simulink model "controller"  (Simulink 7.8)
settings: Solver=FixedStepDiscrete  SolverMode=SingleTasking  StartTime=0.0  StopTime=10.0  FixedStep=0.01  RelTol=1e-3
InitFcn:
  | Busses
  | missions
  | common
  | physical_constants
  | l2plus
model workspace: external: MATLAB File (data not in the file)
values from neighbouring files (symbols this model uses):
  InitialPoint = 0    [l2plus.m]
  IPStar = 0    [l2plus.m]
  lla_ltp_gain = [r * (pi / 180 / 1e7); v * cos(ref_lla(1)) * (pi / 180 / 1e7); 1e-6]    [common.m]
  MaxDwnPthStar = 1    [l2plus.m]
  switchDistance = 4    [l2plus.m]
  T_step = 0.01    [common.m]
  tanIntercept = tan( 45*pi/180 )    [l2plus.m]
  TStar = single(2)    [l2plus.m]
  Turn2Track = 0    [l2plus.m]
  wheelbase = 3.27    [physical_constants.m]
undefined symbols (not defined in the file or in its folder): DiscIntNeverNeededParam, gps_offset, GpsOffsetCorrectionEnable, gpsOrigin, KPsiDot, test_waypoints
libraries: uSimLib x16, aerolibutil x2, aerolibtransform2 x1
settings Model: Creator=bwmairs  LastModifiedBy=Bryant
settings DataIOCC: SignalLogging=off  DSMLogging=off
settings OptimizationCC: BlockReduction=off  InlineParams=on  InlineInvariantSignals=on  PassReuseOutputArgsAs=Individual arguments  ZeroExternalMemoryAtStartup=off  ZeroInternalMemoryAtStartup=off  InitFltsAndDblsToZero=on  NoFixptDivByZeroProtection=on  EfficientFloat2IntCast=on  OptimizeModelRefInitCode=on  LifeSpan=30
settings DebuggingCC: ReadBeforeWriteMsg=DisableAll  WriteAfterWriteMsg=DisableAll  WriteAfterReadMsg=DisableAll  UnderspecifiedInitializationDetection=Simplified  ParameterOverflowMsg=warning  FcnCallInpInsideContextMsg=Use local settings  UniqueDataStoreMsg=error
settings HardwareCC: ProdHWDeviceType=Generic->Unspecified (assume 32-bit Generic)  TargetBitPerInt=16  TargetBitPerPointer=16  TargetIntDivRoundTo=Zero  TargetEndianess=LittleEndian  TargetWordSize=16  TargetHWDeviceType=Microchip->dsPIC  ProdEqTarget=off
settings ModelReferenceCC: ModelReferenceNumInstancesAllowed=Single
settings SFSimCC: SimCustomHeaderCode="#include \"Missions.h\""  SimUserIncludeDirs=../Libs/C  SimParseCustomCode=off
settings RTWCC: SystemTargetFile=ert.tlc  GenCodeOnly=on  GenerateMakefile=off  TemplateMakefile=ert_default_tmf  Description=Embedded Coder  ProcessScript=ert_make_rtw_hook  RTWCompilerOptimization=On
settings CodeAppCC: IgnoreCustomStorageClasses=off  IgnoreTestpoints=on
settings ERTTargetCC: MultiwordLength=2048  IncludeMdlTerminateFcn=off  SupportComplex=off  InlinedParameterPlacement=NonHierarchical  ERTCustomFileTemplate=example_file_process.tlc  ConvertIfToSwitch=off  SuppressUnreachableDefaultCases=off

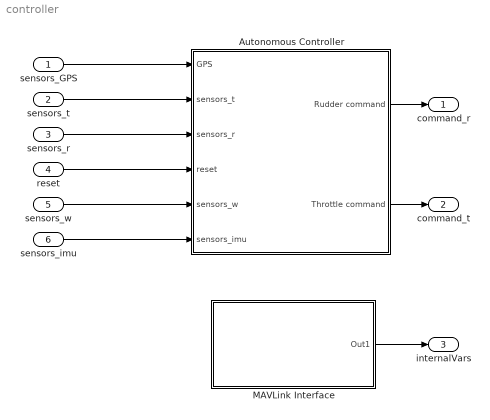
== system controller ==
  sensors_GPS : Inport  OutDataTypeStr=Bus: GpsData  PortDimensions=1
  sensors_t : Inport  Port=2  OutDataTypeStr=int16  PortDimensions=1
  sensors_r : Inport  Port=3  OutDataTypeStr=single  PortDimensions=1
  reset : Inport  Port=4  OutDataTypeStr=boolean  PortDimensions=1
  sensors_w : Inport  Port=5  OutDataTypeStr=single  PortDimensions=1
  sensors_imu : Inport  Port=6  OutDataTypeStr=Bus: ImuData  PortDimensions=1
  Autonomous Controller : Subsystem  Priority=1
  MAVLink Interface : Subsystem
  command_r : Outport  OutDataTypeStr=single  PortDimensions=1
  command_t : Outport  Port=2  OutDataTypeStr=int16  PortDimensions=1
  internalVars : Outport  Port=3  OutDataTypeStr=Bus: InternalVariables  PortDimensions=1
  wires:
  sensors_t/1 -> Autonomous Controller/2(sensors_t)
  sensors_GPS/1 -> Autonomous Controller/1(GPS)
  reset/1 -> Autonomous Controller/4(reset)
  sensors_r/1 -> Autonomous Controller/3(sensors_r)
  Autonomous Controller/2(Throttle command) -> command_t/1
  Autonomous Controller/1(Rudder command) -> command_r/1
  sensors_w/1 -> Autonomous Controller/5(sensors_w)
  MAVLink Interface/1(Out1) -> internalVars/1
  sensors_imu/1 -> Autonomous Controller/6(sensors_imu)

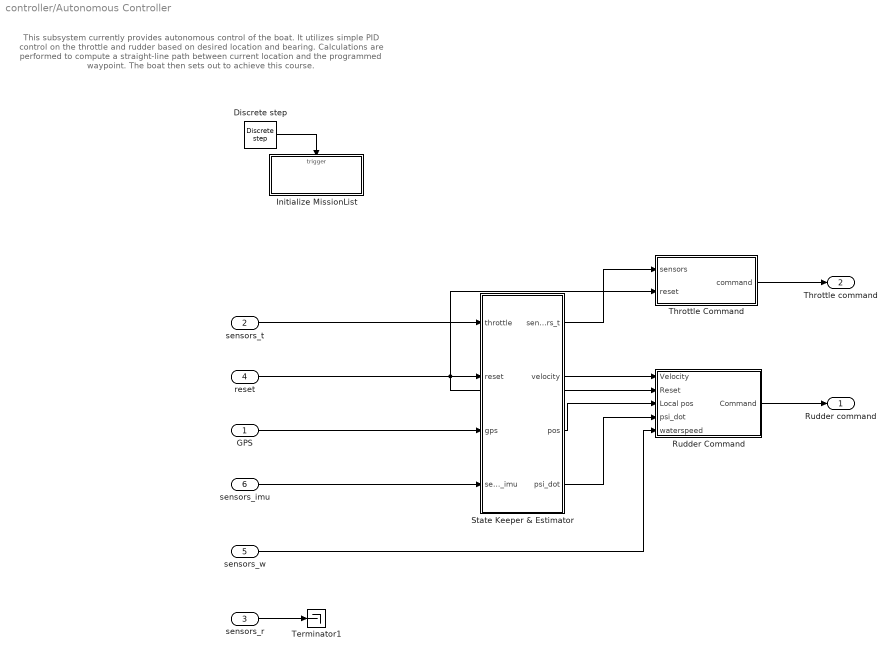
== system controller/Autonomous Controller ==
  note: This subsystem currently provides autonomous control of the boat. It utilizes simple PID control
      | on the throttle and rudder based on desired location and bearing. Calculations are performed
      | to compute a straight-line path between current location and the programmed waypoint. The
      | boat then sets out to achieve this course.
  GPS : Inport
  sensors_t : Inport  Port=2
  sensors_r : Inport  Port=3
  reset : Inport  Port=4
  sensors_w : Inport  Port=5
  sensors_imu : Inport  Port=6
  Discrete step : uSimLib/Sources/Discrete step  start_value=1  end_value=0  transition_time=1
  Initialize MissionList : Subsystem  TreatAsAtomicUnit=on
  Rudder Command : Subsystem
  State Keeper & Estimator : Subsystem
  Terminator1 : Terminator
  Throttle Command : Subsystem
  Rudder command : Outport
  Throttle command : Outport  Port=2
  wires:
  Discrete step/1 -> Initialize MissionList/Trigger
  reset/1 -> Rudder Command/2(Reset), Throttle Command/2(reset), State Keeper & Estimator/2(reset)
  State Keeper & Estimator/3(pos) -> Rudder Command/3(Local pos)
  State Keeper & Estimator/1(sensors_t) -> Throttle Command/1(sensors)
  State Keeper & Estimator/2(velocity) -> Rudder Command/1(Velocity)
  GPS/1 -> State Keeper & Estimator/3(gps)
  Throttle Command/1(command) -> Throttle command/1
  Rudder Command/1(Command) -> Rudder command/1
  sensors_r/1 -> Terminator1/1
  sensors_t/1 -> State Keeper & Estimator/1(throttle)
  State Keeper & Estimator/4(psi_dot) -> Rudder Command/4(psi_dot)
  sensors_w/1 -> Rudder Command/5(waterspeed)
  sensors_imu/1 -> State Keeper & Estimator/4(sensors_imu)

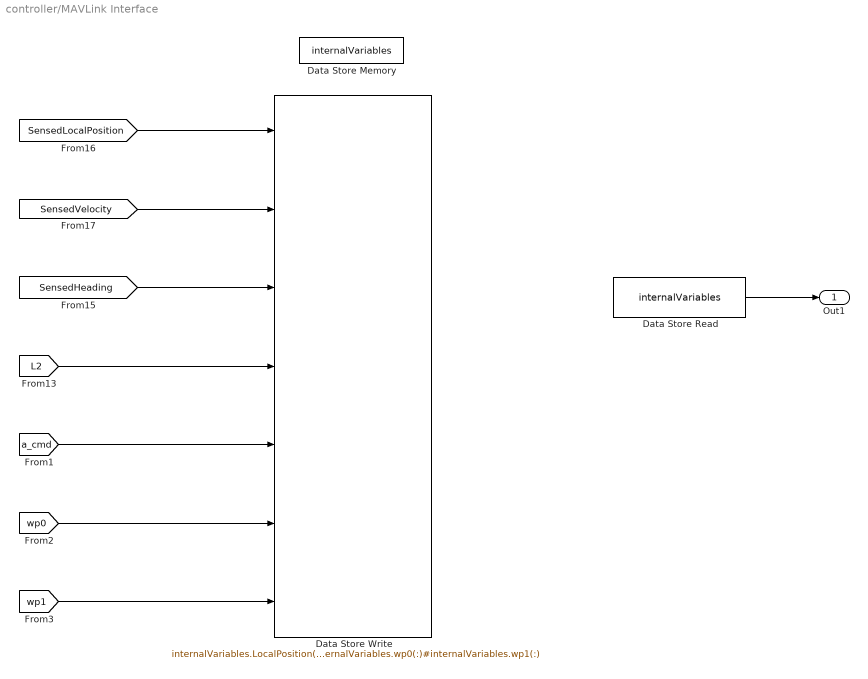
== system controller/MAVLink Interface ==
  Data Store Memory : DataStoreMemory  DataStoreName=internalVariables  OutDataTypeStr=Bus: InternalVariables
  Data Store Read : DataStoreRead  DataStoreName=internalVariables  SampleTime=T_step  DataStoreElements=internalVariables
  Data Store Write : DataStoreWrite  DataStoreName=internalVariables  DataStoreElements=internalVariables.LocalPosition(:)#internalVariables.Velocity(:)#internalVariables.Heading#internalVariables.L2Vector(:)#internalVariables.Acmd#internalVariables.wp0(:)#internalVariables.wp1(:)
  Out1 : Outport  OutDataTypeStr=Bus: InternalVariables
  wires:
  [SensedLocalPosition] -> Data Store Write/1
  [SensedVelocity] -> Data Store Write/2
  [SensedHeading] -> Data Store Write/3
  [L2] -> Data Store Write/4
  [a_cmd] -> Data Store Write/5
  [wp0] -> Data Store Write/6
  [wp1] -> Data Store Write/7
  Data Store Read/1 -> Out1/1

== system controller/Autonomous Controller/Initialize MissionList ==
  Trigger : TriggerPort  TriggerType=falling  PortDimensions=1
  AppendMission : uSimLib/Mission Manager/AppendMission  Priority=-2  sampleTime=-1
  ClearMissionList : uSimLib/Mission Manager/ClearMissionList  Priority=-1  sampleTime=-1
  Constant : Constant  Value=test_waypoints(1)  OutDataTypeStr=Bus: Mission
  Data Type Conversion : DataTypeConversion  OutDataTypeStr=uint8  RndMeth=Simplest
  Mission Init : uSimLib/Mission Manager/Mission Init  Priority=-3  maxMissions=16  sampleTime=-1
  Mission InitAll : uSimLib/Mission Manager/Mission InitAll  Priority=0  maxMissions=16  sampleTime=-1  missionsVar=test_waypoints
  SetCurrentMission : uSimLib/Mission Manager/SetCurrentMission  sampleTime=-1
  wires:
  AppendMission/1 -> Data Type Conversion/1
  Constant/1 -> AppendMission/1
  Data Type Conversion/1 -> SetCurrentMission/1

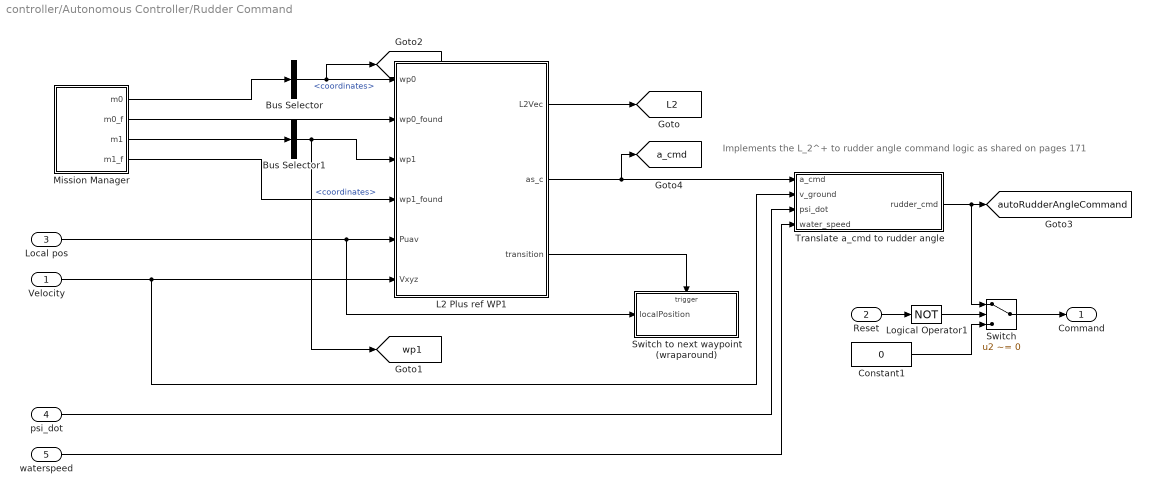
== system controller/Autonomous Controller/Rudder Command ==
  note: Implements the L_2^+ to rudder angle command logic as shared on pages 171
  Velocity : Inport
  Reset : Inport  Port=2
  Local pos : Inport  Port=3
  psi_dot : Inport  Port=4
  waterspeed : Inport  Port=5
  Bus Selector : BusSelector  OutputSignals=coordinates
  Bus Selector1 : BusSelector  OutputSignals=coordinates
  Constant1 : Constant  Value=0  OutDataTypeStr=single
  L2 Plus ref WP1 : MATLAB Function  TreatAsAtomicUnit=on
  Logical Operator1 : Logic  Operator=NOT  Inputs=1  AllPortsSameDT=off  OutDataTypeStr=boolean
  Mission Manager : Subsystem
  Switch : Switch  Criteria=u2 ~= 0
  Switch to next waypoint (wraparound) : Subsystem  TreatAsAtomicUnit=on
  Translate a_cmd to rudder angle : Subsystem
  Command : Outport
  tag scope: L2=global, a_cmd=global, autoRudderAngleCommand=global, wp0=global, wp1=global
  wires:
  Bus Selector1/1 -> L2 Plus ref WP1/3(wp1), [wp1]  "<coordinates>"
  Bus Selector/1 -> [wp0], L2 Plus ref WP1/1(wp0)  "<coordinates>"
  Mission Manager/1(m0) -> Bus Selector/1
  Mission Manager/2(m0_f) -> L2 Plus ref WP1/2(wp0_found)
  L2 Plus ref WP1/3(transition) -> Switch to next waypoint (wraparound)/Trigger
  Mission Manager/4(m1_f) -> L2 Plus ref WP1/4(wp1_found)
  Mission Manager/3(m1) -> Bus Selector1/1
  Local pos/1 -> Switch to next waypoint (wraparound)/1(localPosition), L2 Plus ref WP1/5(Puav)
  Velocity/1 -> L2 Plus ref WP1/6(Vxyz), Translate a_cmd to rudder angle/2(v_ground)
  L2 Plus ref WP1/1(L2Vec) -> [L2]
  Translate a_cmd to rudder angle/1(rudder_cmd) -> [autoRudderAngleCommand], Switch/1
  Reset/1 -> Logical Operator1/1
  Logical Operator1/1 -> Switch/2
  L2 Plus ref WP1/2(as_c) -> [a_cmd], Translate a_cmd to rudder angle/1(a_cmd)
  psi_dot/1 -> Translate a_cmd to rudder angle/3(psi_dot)
  waterspeed/1 -> Translate a_cmd to rudder angle/4(water_speed)
  Constant1/1 -> Switch/3
  Switch/1 -> Command/1

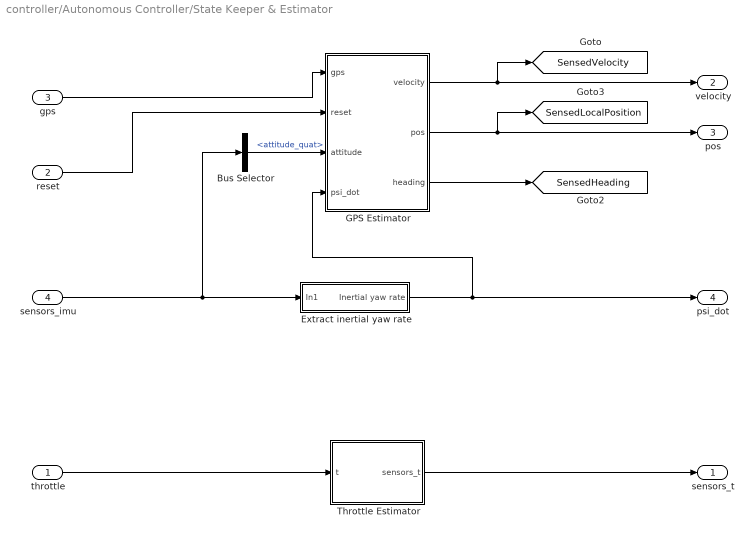
== system controller/Autonomous Controller/State Keeper & Estimator ==
  throttle : Inport
  reset : Inport  Port=2
  gps : Inport  Port=3
  sensors_imu : Inport  Port=4
  Bus Selector : BusSelector  OutputSignals=attitude_quat
  Extract inertial yaw rate : Subsystem
  GPS Estimator : Subsystem
  Throttle Estimator : Subsystem
  sensors_t : Outport
  velocity : Outport  Port=2
  pos : Outport  Port=3
  psi_dot : Outport  Port=4
  tag scope: SensedHeading=global, SensedLocalPosition=global, SensedVelocity=global
  wires:
  Throttle Estimator/1(sensors_t) -> sensors_t/1
  GPS Estimator/3(heading) -> [SensedHeading]
  GPS Estimator/2(pos) -> [SensedLocalPosition], pos/1
  gps/1 -> GPS Estimator/1(gps)
  GPS Estimator/1(velocity) -> [SensedVelocity], velocity/1
  reset/1 -> GPS Estimator/2(reset)
  throttle/1 -> Throttle Estimator/1(t)
  sensors_imu/1 -> Extract inertial yaw rate/1(In1), Bus Selector/1
  Extract inertial yaw rate/1(Inertial yaw rate) -> psi_dot/1, GPS Estimator/4(psi_dot)
  Bus Selector/1 -> GPS Estimator/3(attitude)  "<attitude_quat>"

== system controller/Autonomous Controller/Throttle Command ==
  sensors : Inport
  reset : Inport  Port=2
  Constant1 : Constant  Value=0  OutDataTypeStr=int16
  Constant5 : Constant  Value=1000  OutDataTypeStr=int16
  Switch : Switch  Criteria=u2 > Threshold
  Terminator : Terminator
  command : Outport
  tag scope: autoThrottleCommand=global
  wires:
  Constant5/1 -> Switch/3
  Constant1/1 -> Switch/1
  reset/1 -> Switch/2
  sensors/1 -> Terminator/1
  Switch/1 -> [autoThrottleCommand], command/1

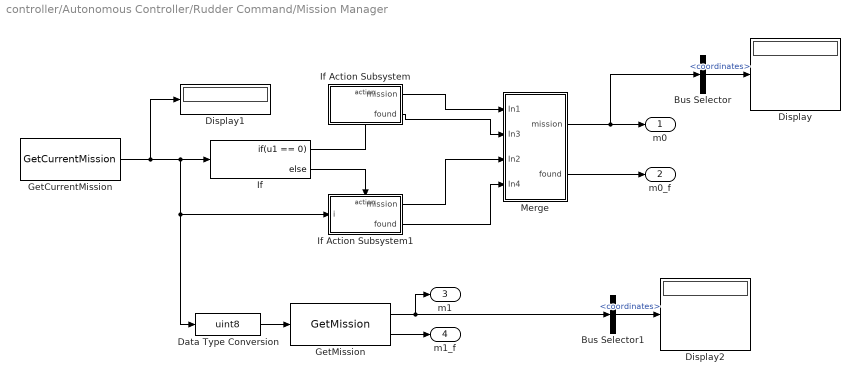
== system controller/Autonomous Controller/Rudder Command/Mission Manager ==
  Bus Selector : BusSelector  OutputSignals=coordinates
  Bus Selector1 : BusSelector  OutputSignals=coordinates
  Data Type Conversion : DataTypeConversion  OutDataTypeStr=uint8
  Display : Display
  Display1 : Display
  Display2 : Display
  GetCurrentMission : uSimLib/Mission Manager/GetCurrentMission  sampleTime=T_step
  GetMission : uSimLib/Mission Manager/GetMission  sampleTime=T_step
  If : If  IfExpression=u1 == 0
  If Action Subsystem : Subsystem  TreatAsAtomicUnit=on
  If Action Subsystem1 : Subsystem  TreatAsAtomicUnit=on
  Merge : Subsystem
  m0 : Outport
  m0_f : Outport  Port=2
  m1 : Outport  Port=3
  m1_f : Outport  Port=4
  wires:
  Data Type Conversion/1 -> GetMission/1
  Merge/2(found) -> m0_f/1
  Merge/1(mission) -> m0/1, Bus Selector/1
  If Action Subsystem1/2(found) -> Merge/4(In4)
  If Action Subsystem/2(found) -> Merge/2(In3)
  If Action Subsystem1/1(mission) -> Merge/3(In2)
  If Action Subsystem/1(mission) -> Merge/1(In1)
  If/2 -> If Action Subsystem1/Action
  If/1 -> If Action Subsystem/Action
  GetMission/2 -> m1_f/1
  GetMission/1 -> m1/1, Bus Selector1/1
  GetCurrentMission/1 -> If/1, Data Type Conversion/1, If Action Subsystem1/1(i), Display1/1
  Bus Selector/1 -> Display/1  "<coordinates>"
  Bus Selector1/1 -> Display2/1  "<coordinates>"

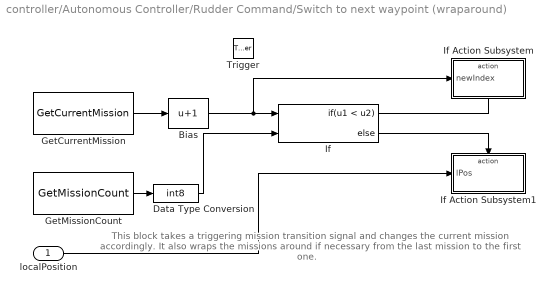
== system controller/Autonomous Controller/Rudder Command/Switch to next waypoint (wraparound) ==
  note: This block takes a triggering mission transition signal
      | and changes the current mission accordingly. It also
      | wraps the missions around if necessary from the last
      | mission to the first one.
  localPosition : Inport
  Trigger : TriggerPort
  Bias : Bias  Bias=1
  Data Type Conversion : DataTypeConversion  OutDataTypeStr=int8
  GetCurrentMission : uSimLib/Mission Manager/GetCurrentMission  sampleTime=-1
  GetMissionCount : uSimLib/Mission Manager/GetMissionCount  sampleTime=-1
  If : If  NumInputs=2  IfExpression=u1 < u2
  If Action Subsystem : Subsystem  TreatAsAtomicUnit=on
  If Action Subsystem1 : Subsystem  TreatAsAtomicUnit=on
  wires:
  Data Type Conversion/1 -> If/2
  If/2 -> If Action Subsystem1/Action
  If/1 -> If Action Subsystem/Action
  Bias/1 -> If/1, If Action Subsystem/1(newIndex)
  GetMissionCount/1 -> Data Type Conversion/1
  GetCurrentMission/1 -> Bias/1
  localPosition/1 -> If Action Subsystem1/1(lPos)

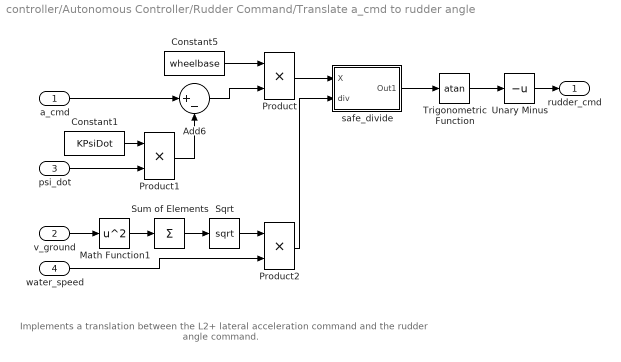
== system controller/Autonomous Controller/Rudder Command/Translate a_cmd to rudder angle ==
  note: Implements a translation between the L2+ lateral acceleration command
      | and the rudder angle command.
  a_cmd : Inport
  v_ground : Inport  Port=2
  psi_dot : Inport  Port=3
  water_speed : Inport  Port=4
  Add6 : Sum  Inputs=|+-
  Constant1 : Constant  Value=KPsiDot
  Constant5 : Constant  Value=wheelbase
  Math Function1 : Math  Operator=square  SaturateOnIntegerOverflow=on
  Product : Product  Inputs=**  RndMeth=Zero
  Product1 : Product  Inputs=**  RndMeth=Zero
  Product2 : Product  Inputs=**  RndMeth=Zero
  Sqrt : Sqrt  SaturateOnIntegerOverflow=on
  Sum of Elements : Sum  Inputs=+
  Trigonometric Function : Trigonometry  Operator=atan
  Unary Minus : UnaryMinus
  safe_divide : Subsystem  TreatAsAtomicUnit=on
      settings: RTWFcnNameOpts=Use subsystem name  RTWFileNameOpts=Use function name
  rudder_cmd : Outport
  wires:
  Constant5/1 -> Product/1
  Product/1 -> safe_divide/1(X)
  Trigonometric Function/1 -> Unary Minus/1
  Math Function1/1 -> Sum of Elements/1
  Sum of Elements/1 -> Sqrt/1
  safe_divide/1(Out1) -> Trigonometric Function/1
  Add6/1 -> Product/2
  v_ground/1 -> Math Function1/1
  Unary Minus/1 -> rudder_cmd/1
  a_cmd/1 -> Add6/1
  psi_dot/1 -> Product1/2
  Constant1/1 -> Product1/1
  Sqrt/1 -> Product2/1
  Product2/1 -> safe_divide/2(div)
  water_speed/1 -> Product2/2
  Product1/1 -> Add6/2

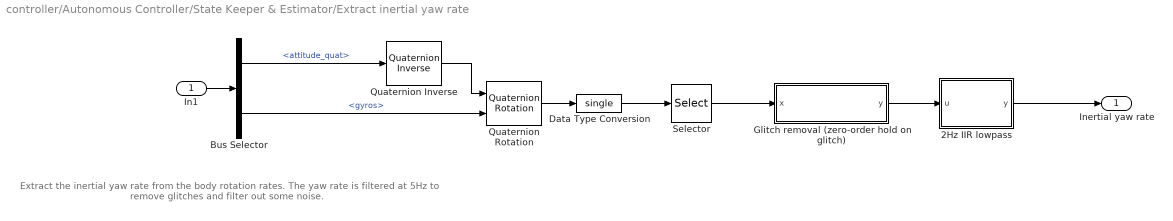
== system controller/Autonomous Controller/State Keeper & Estimator/Extract inertial yaw rate ==
  note: Extract the inertial yaw rate from the body rotation rates.
      | The yaw rate is filtered at 5Hz to remove glitches and filter out some noise.
  In1 : Inport
  2Hz IIR lowpass : MATLAB Function  TreatAsAtomicUnit=on
  Bus Selector : BusSelector  OutputSignals=attitude_quat,gyros
  Data Type Conversion : DataTypeConversion  OutDataTypeStr=single
  Glitch removal (zero-order hold on glitch) : MATLAB Function  TreatAsAtomicUnit=on
  Quaternion Inverse : aerolibutil/Quaternion Inverse
  Quaternion Rotation : aerolibutil/Quaternion Rotation
  Selector : Selector  InputPortWidth=3  IndexOptions=Index vector (dialog)  Indices=[3]  OutputSizes=1
  Inertial yaw rate : Outport
  wires:
  In1/1 -> Bus Selector/1
  Quaternion Inverse/1 -> Quaternion Rotation/1
  Quaternion Rotation/1 -> Data Type Conversion/1
  Data Type Conversion/1 -> Selector/1
  Selector/1 -> Glitch removal (zero-order hold on glitch)/1(x)
  Glitch removal (zero-order hold on glitch)/1(y) -> 2Hz IIR lowpass/1(u)
  Bus Selector/2 -> Quaternion Rotation/2  "<gyros>"
  2Hz IIR lowpass/1(y) -> Inertial yaw rate/1
  Bus Selector/1 -> Quaternion Inverse/1  "<attitude_quat>"

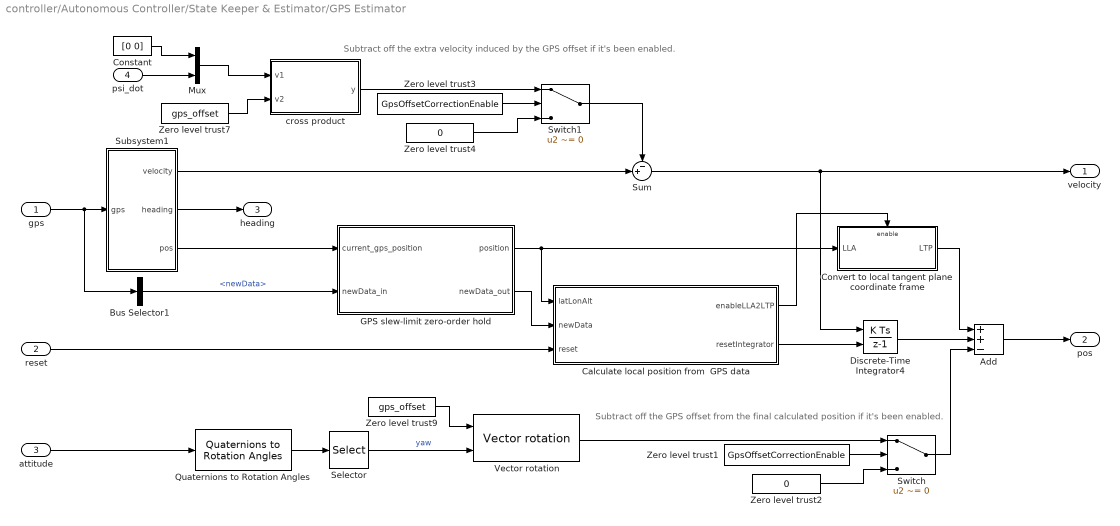
== system controller/Autonomous Controller/State Keeper & Estimator/GPS Estimator ==
  note: Subtract off the GPS offset from the final calculated position if it's
      | been enabled.
  note: Subtract off the extra velocity induced by the GPS offset
      | if it's been enabled.
  gps : Inport
  reset : Inport  Port=2
  attitude : Inport  Port=3
  psi_dot : Inport  Port=4  OutDataTypeStr=single
  Add : Sum  Inputs=++-
  Bus Selector1 : BusSelector  OutputSignals=newData
  Calculate local position from  GPS data : MATLAB Function  TreatAsAtomicUnit=on
  Constant : Constant  Value=[0 0]  OutDataTypeStr=single
  Convert to local tangent plane coordinate frame : Subsystem  TreatAsAtomicUnit=on  RTWFcnName=lla2ltp
      settings: RTWFcnNameOpts=User specified
  Discrete-Time Integrator4 : DiscreteIntegrator  ExternalReset=level  SampleTime=-1  ICPrevOutput=DiscIntNeverNeededParam  ICPrevScaledInput=DiscIntNeverNeededParam
  GPS slew-limit zero-order hold : MATLAB Function  TreatAsAtomicUnit=on
  Mux : Mux  Inputs=2
  Quaternions to Rotation Angles : aerolibtransform2/Quaternions to Rotation Angles  rotationOrder=ZYX
  Selector : Selector  InputPortWidth=3  IndexOptions=Index vector (dialog)  Indices=[1]  OutputSizes=1
  Subsystem1 : Subsystem
  Sum : Sum  Inputs=-+|
  Switch : Switch  Criteria=u2 ~= 0  OutDataTypeStr=Inherit: Inherit via back propagation  RndMeth=Simplest
  Switch1 : Switch  Criteria=u2 ~= 0  OutDataTypeStr=Inherit: Inherit via back propagation  RndMeth=Simplest
  Vector rotation : uSimLib/Math/Vector rotation
  Zero level trust1 : Constant  Value=GpsOffsetCorrectionEnable  OutDataTypeStr=boolean
  Zero level trust2 : Constant  Value=0  OutDataTypeStr=single
  Zero level trust3 : Constant  Value=GpsOffsetCorrectionEnable  OutDataTypeStr=boolean
  Zero level trust4 : Constant  Value=0  OutDataTypeStr=single
  Zero level trust7 : Constant  Value=gps_offset  OutDataTypeStr=single
  Zero level trust9 : Constant  Value=gps_offset  OutDataTypeStr=single
  cross product : MATLAB Function  TreatAsAtomicUnit=on
  velocity : Outport
  pos : Outport  Port=2
  heading : Outport  Port=3
  wires:
  Calculate local position from  GPS data/2(resetIntegrator) -> Discrete-Time Integrator4/2
  Add/1 -> pos/1
  Discrete-Time Integrator4/1 -> Add/2
  Subsystem1/3(pos) -> GPS slew-limit zero-order hold/1(current_gps_position)
  gps/1 -> Bus Selector1/1, Subsystem1/1(gps)
  Subsystem1/2(heading) -> heading/1
  reset/1 -> Calculate local position from  GPS data/3(reset)
  Convert to local tangent plane coordinate frame/1(LTP) -> Add/1
  Calculate local position from  GPS data/1(enableLLA2LTP) -> Convert to local tangent plane coordinate frame/Enable
  GPS slew-limit zero-order hold/1(position) -> Calculate local position from  GPS data/1(latLonAlt), Convert to local tangent plane coordinate frame/1(LLA)
  GPS slew-limit zero-order hold/2(newData_out) -> Calculate local position from  GPS data/2(newData)
  Bus Selector1/1 -> GPS slew-limit zero-order hold/2(newData_in)  "<newData>"
  attitude/1 -> Quaternions to Rotation Angles/1
  Quaternions to Rotation Angles/1 -> Selector/1
  Constant/1 -> Mux/1
  psi_dot/1 -> Mux/2
  Zero level trust7/1 -> cross product/2(v2)
  Mux/1 -> cross product/1(v1)
  Subsystem1/1(velocity) -> Sum/2
  Sum/1 -> Discrete-Time Integrator4/1, velocity/1
  Selector/1 -> Vector rotation/2  "yaw"
  Zero level trust9/1 -> Vector rotation/1
  cross product/1(y) -> Switch1/1
  Switch/1 -> Add/3
  Zero level trust1/1 -> Switch/2
  Vector rotation/1 -> Switch/1
  Zero level trust2/1 -> Switch/3
  Zero level trust3/1 -> Switch1/2
  Zero level trust4/1 -> Switch1/3
  Switch1/1 -> Sum/1

== system controller/Autonomous Controller/State Keeper & Estimator/Throttle Estimator ==
  t : Inport
  sensors_t : Outport
  wires:
  t/1 -> sensors_t/1

== system controller/Autonomous Controller/Rudder Command/Mission Manager/If Action Subsystem ==
  Action Port : ActionPort  ActionType=then
  Constant : Constant  Value=true  OutDataTypeStr=boolean
  GetStartingPoint : uSimLib/Mission Manager/GetStartingPoint  sampleTime=-1
  mission : Outport
  found : Outport  Port=2
  wires:
  Constant/1 -> found/1
  GetStartingPoint/1 -> mission/1

== system controller/Autonomous Controller/Rudder Command/Mission Manager/If Action Subsystem1 ==
  i : Inport
  Action Port : ActionPort  ActionType=else
  Bias : Bias  Bias=-1
  Data Type Conversion : DataTypeConversion  OutDataTypeStr=uint8
  GetMission : uSimLib/Mission Manager/GetMission  sampleTime=-1
  mission : Outport
  found : Outport  Port=2
  wires:
  Data Type Conversion/1 -> GetMission/1
  Bias/1 -> Data Type Conversion/1
  GetMission/2 -> found/1
  i/1 -> Bias/1
  GetMission/1 -> mission/1

== system controller/Autonomous Controller/Rudder Command/Mission Manager/Merge ==
  In1 : Inport
  In3 : Inport  Port=2
  In2 : Inport  Port=3
  In4 : Inport  Port=4
  Merge : Merge
  Merge1 : Merge
  mission : Outport
  found : Outport  Port=2
  wires:
  In4/1 -> Merge1/2
  Merge1/1 -> found/1
  In3/1 -> Merge1/1
  In2/1 -> Merge/2
  Merge/1 -> mission/1
  In1/1 -> Merge/1

== system controller/Autonomous Controller/Rudder Command/Switch to next waypoint (wraparound)/If Action Subsystem ==
  newIndex : Inport
  Action Port : ActionPort  ActionType=then
  Data Type Conversion : DataTypeConversion  OutDataTypeStr=uint8
  SetCurrentMission : uSimLib/Mission Manager/SetCurrentMission  sampleTime=-1
  wires:
  Data Type Conversion/1 -> SetCurrentMission/1
  newIndex/1 -> Data Type Conversion/1

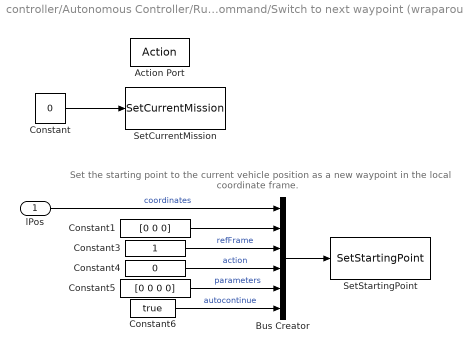
== system controller/Autonomous Controller/Rudder Command/Switch to next waypoint (wraparound)/If Action Subsystem1 ==
  note: Set the starting point to the current vehicle position as a new waypoint in the local coordinate frame.
  lPos : Inport
  Action Port : ActionPort  ActionType=else
  Bus Creator : BusCreator  Inputs=6  OutDataTypeStr=Bus: Mission  NonVirtualBus=on
  Constant : Constant  Value=0  OutDataTypeStr=uint8
  Constant1 : Constant  Value=[0 0 0]  OutDataTypeStr=single
  Constant3 : Constant  OutDataTypeStr=uint8
  Constant4 : Constant  Value=0  OutDataTypeStr=uint8
  Constant5 : Constant  Value=[0 0 0 0]  OutDataTypeStr=single
  Constant6 : Constant  Value=true  OutDataTypeStr=boolean
  SetCurrentMission : uSimLib/Mission Manager/SetCurrentMission  sampleTime=-1
  SetStartingPoint : uSimLib/Mission Manager/SetStartingPoint  sampleTime=-1
  wires:
  Constant/1 -> SetCurrentMission/1
  Constant6/1 -> Bus Creator/6  "autocontinue"
  Constant5/1 -> Bus Creator/5  "parameters"
  Constant4/1 -> Bus Creator/4  "action"
  Constant3/1 -> Bus Creator/3  "refFrame"
  lPos/1 -> Bus Creator/1  "coordinates"
  Bus Creator/1 -> SetStartingPoint/1
  Constant1/1 -> Bus Creator/2

== system controller/Autonomous Controller/Rudder Command/Translate a_cmd to rudder angle/safe_divide ==
  X : Inport
  div : Inport  Port=2
  Constant1 : Constant  Value=0  OutDataTypeStr=Inherit: Inherit via back propagation
  Product : Product  Inputs=*/  RndMeth=Zero
  Switch : Switch  Criteria=u2 ~= 0
  Out1 : Outport
  wires:
  X/1 -> Product/1
  div/1 -> Product/2, Switch/2
  Product/1 -> Switch/1
  Constant1/1 -> Switch/3
  Switch/1 -> Out1/1

== system controller/Autonomous Controller/State Keeper & Estimator/GPS Estimator/Convert to local tangent plane coordinate frame ==
  LLA : Inport
  Enable : EnablePort
  LLA2LTP : Subsystem  TreatAsAtomicUnit=on  RTWFcnName=lla2ltp
      settings: RTWFcnNameOpts=User specified
  LTP : Outport  OutDataTypeStr=single  InitialOutput=[0, 0, 0]
  wires:
  LLA/1 -> LLA2LTP/1(LLA)
  LLA2LTP/1(LTP) -> LTP/1

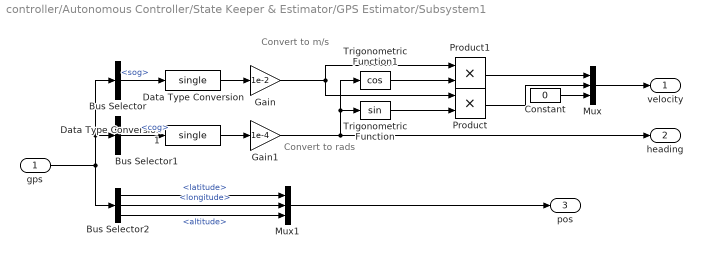
== system controller/Autonomous Controller/State Keeper & Estimator/GPS Estimator/Subsystem1 ==
  note: Convert to m/s
  note: Convert to rads
  gps : Inport
  Bus Selector : BusSelector  OutputSignals=sog
  Bus Selector1 : BusSelector  OutputSignals=cog
  Bus Selector2 : BusSelector  OutputSignals=latitude,longitude,altitude
  Constant : Constant  Value=0  OutDataTypeStr=single
  Data Type Conversion : DataTypeConversion  OutDataTypeStr=single  RndMeth=Simplest
  Data Type Conversion1 : DataTypeConversion  OutDataTypeStr=single  RndMeth=Simplest
  Gain : Gain  Gain=1e-2
  Gain1 : Gain  Gain=1e-4
  Mux : Mux  Inputs=3
  Mux1 : Mux  Inputs=3
  Product : Product  OutDataTypeStr=single  RndMeth=Zero
  Product1 : Product  OutDataTypeStr=single  RndMeth=Zero
  Trigonometric Function : Trigonometry
  Trigonometric Function1 : Trigonometry  Operator=cos
  velocity : Outport
  heading : Outport  Port=2
  pos : Outport  Port=3
  wires:
  gps/1 -> Bus Selector/1, Bus Selector1/1, Bus Selector2/1
  Bus Selector1/1 -> Data Type Conversion1/1  "<cog>"
  Trigonometric Function/1 -> Product/2
  Trigonometric Function1/1 -> Product1/2
  Product1/1 -> Mux/1
  Product/1 -> Mux/2
  Constant/1 -> Mux/3
  Mux/1 -> velocity/1
  Bus Selector/1 -> Data Type Conversion/1  "<sog>"
  Bus Selector2/2 -> Mux1/2  "<longitude>"
  Bus Selector2/3 -> Mux1/3  "<altitude>"
  Mux1/1 -> pos/1
  Bus Selector2/1 -> Mux1/1  "<latitude>"
  Data Type Conversion/1 -> Gain/1
  Data Type Conversion1/1 -> Gain1/1
  Gain/1 -> Product1/1, Product/1
  Gain1/1 -> heading/1, Trigonometric Function/1, Trigonometric Function1/1

== system controller/Autonomous Controller/State Keeper & Estimator/GPS Estimator/Convert to local tangent plane coordinate frame/LLA2LTP ==
  LLA : Inport
  Add : Sum  Inputs=+-  OutDataTypeStr=single  RndMeth=Simplest  InputSameDT=on
  Constant : Constant  Value=gpsOrigin  OutDataTypeStr=int32
  Constant1 : Constant  Value=lla_ltp_gain  OutDataTypeStr=single
  Product : Product  OutDataTypeStr=single  RndMeth=Simplest  LockScale=on
  LTP : Outport  OutDataTypeStr=single  InitialOutput=[0, 0, 0]
  wires:
  Add/1 -> Product/1
  Constant1/1 -> Product/2
  Product/1 -> LTP/1
  Constant/1 -> Add/2
  LLA/1 -> Add/1

== matlab function Autonomous Controller/State Keeper & Estimator/GPS Estimator/cross product ==
  data: v1 input double size=3; y output double; v2 input double size=3
function y = cross_product(v1, v2)
%#codegen
    i = (v1(2) * v2(3) - v2(2) * v1(3));
    j = (v1(3) * v2(1) - v2(3) * v1(1));
    k = (v1(1) * v2(2) - v2(1) * v1(2));
    y = [i, j, k];
end

== matlab function Autonomous Controller/State Keeper & Estimator/GPS Estimator/GPS slew-limit zero-order hold ==
  data: position output int32 size=3; current_gps_position input int32 size=3; newData_in input boolean size=1; gps_leap_rate_limit parameter int32 size=1; newData_out output double
function [position, newData_out] = limit_gps_rate(current_gps_position, newData_in, gps_leap_rate_limit)
%% This function enforces a slew cap on the GPS data by straight-up removing
% outliers based on a given `gps_leap_rate_limit` value. 
% first_datapoint - Boolean for whether this is the first valid GPS fix.
% gps_leap_rate_limit - a value in degrees as to how fast the GPS position can
%                       change in a single timestep
% Outputs:
% position - The filtered GPS position
% valid - Whether this is a new value.

% Store the last GPS location, used for derivative calculations
persistent last_gps_position last_timestep current_timestep firstDataPoint;
if isempty(last_gps_position)
    last_gps_position = current_gps_position;
    current_timestep = int32(0);
    last_timestep = int32(0);
    firstDataPoint = true;
end

% If this is the first data point, latch it to begin the slew capping.
if firstDataPoint && newData_in
    last_gps_position = current_gps_position;
    current_timestep = int32(0);
    last_timestep = int32(0);
    firstDataPoint = false;
end

% If the slew limit was exceeded for either the latitude or longitude, only
% output the last timestep. We ignore the altitude completely.
if newData_in && all((current_gps_position - last_gps_position) / (current_timestep - last_timestep) <= gps_leap_rate_limit)
    % Update last timesteps data for future calculations.
    last_gps_position = current_gps_position;
    last_timestep = current_timestep;

    % We can output the current position as it's within the slew limit.
    position = current_gps_position;
    newData_out = true;
else
    position = last_gps_position;
    newData_out = false;
end

% Increment the current timestep handling wrap-arounds nicely. This WILL
% NOT handle situations were the time between valid GPS position updates is
% greater than INT32_MAX, but I can live with that.
if current_timestep == intmax('int32')
    current_timestep = current_timestep - last_timestep;
    last_timestep = int32(0);
else
    current_timestep = current_timestep + int32(1);
end

== matlab function Autonomous Controller/State Keeper & Estimator/GPS Estimator/Calculate local position from GPS data ==
  data: enableLLA2LTP output boolean size=1; latLonAlt input int32 size=3; newData input boolean size=1; reset input boolean size=1; resetIntegrator output boolean size=1
function [enableLLA2LTP, resetIntegrator]  = estimateGPS(latLonAlt, newData, reset)
%#codegen

% This function watches an incoming stream of GPS data and waits for 5
% valid LLA values before it enables LLA to LTP conversion. It also watches
% for updates to a GPS stream in order to reset a velocity integrator for
% position estimation.

% INPUTS:
% latLonAlt - the latitude, longitude, and altitude of the vehicle from GPS
% in radians/meters.
% newData - A boolean signal specifying whether latLonAlt holds new data
% reset - A global reset boolean trigger.

% OUTPUTS:
% enableLLA2LTP - A boolean specifying whether LLA to LTP conversion should
% occur. The only reason it shouldn't is if the GPS hasn't latched valid
% positions yet.
% resetIntegrator - Indicates that the velocity integrator, which is
% calculating position in between GPS fixes, should be reset.

persistent newDataCounter;

% Reset everything on first startup or when a global reset is triggered
if isempty(newDataCounter) || reset
    newDataCounter = uint8(0);
end

% Pass through the global reset to the velocity integrator
if reset
    resetIntegrator = true;
else
    resetIntegrator = false;
end

% Wait for 5 valid GPS inputs before outputting the current position.
% This allows the GPS to stabilize.
if newDataCounter < 5
    if newData && latLonAlt(1) ~= 0 && latLonAlt(2) ~= 0
        newDataCounter = newDataCounter + 1;
    end
    enableLLA2LTP = false;
else
    % Reset the integrator if new data has been received for this timestep
    % as we have a "truth" position now.
    if newData
        resetIntegrator = true;
    end
    enableLLA2LTP = true;
end

== matlab function Autonomous Controller/State Keeper & Estimator/Extract inertial yaw rate/2Hz IIR lowpass ==
  data: u input double; y output single
function y = fcn(u)
%#codegen

persistent y1; % The last output value

if isempty(y1)
    y1 = single(0);
end

h = 0.01; % Set the signal timestep (Tokimec outputs at 100Hz)
T = 1 / 2; % Set the time constant (5Hz in this case)

a = h / (T + h);
y = (1 - a) * y1 + a * u;

% Save the last output value for the next filter iteration
y1 = y;

== matlab function Autonomous Controller/State Keeper & Estimator/Extract inertial yaw rate/Glitch removal (zero-order hold on glitch) ==
  data: y output single size=1; x input single size=1
function y = rate_limited_hold(x)
%% This function enforces a slew-limit on the input signal, using the last
% previous value as its output in these situations

rate_limit = 10; % Rate shouldn't change by more than 10 rads/s in a second

% Store the last datapoin, used for derivative calculations
persistent last_x last_timestep current_timestep firstDataPoint;
if isempty(last_x)
    last_x = x;
    current_timestep = single(0);
    last_timestep = single(0);
    firstDataPoint = true;
end

% If this is the first data point, latch it to begin the slew capping.
if firstDataPoint
    last_x = x;
    current_timestep = single(0);
    last_timestep = single(0);
    firstDataPoint = false;
end

% If the slew limit was exceeded only output the last timestep.
if abs((x - last_x) / (current_timestep - last_timestep)) <= rate_limit
    % Update last timesteps data for future calculations.
    last_x = x;
    last_timestep = current_timestep;

    % We can output the current position as it's within the slew limit.
    y = x;
else
    y = last_x;
end

% Increment the current timestep handling wrap-arounds nicely. We select a
% 4 digit number, which should still be accurate to 0.1.
if current_timestep == single(9999)
    current_timestep = current_timestep - last_timestep;
    last_timestep = single(0);
else
    current_timestep = current_timestep + single(0.01);
end

== matlab function Autonomous Controller/Rudder Command/L2 Plus ref WP1 ==
  data: wp0 input single size=3; wp0_found input boolean size=1; wp1 input single size=3; wp1_found input boolean size=1; L2Vec output single size=3; Puav input single size=3; Vxyz input single size=3; switchDistance parameter double size=1; tanIntercept parameter double size=1; MaxDwnPthStar parameter double size=1; Turn2Track parameter double size=1; InitialPoint parameter double size=1; IPStar parameter double size=1; TStar parameter double size=1; as_c output single size=1; transition output boolean size=1
function [L2Vec, as_c, transition] = L2PlusWP1(wp0, wp0_found, wp1, wp1_found, Puav, Vxyz, switchDistance, ...
    tanIntercept, MaxDwnPthStar,Turn2Track,...
    InitialPoint, IPStar, TStar)
%==============================
%     computes bank angle command for following a straight line
%     by creating an aim point that may be more than L2 away 
%     from the UAV. The aim point is (usually) farther along the path 
%     toward wp1 than the UAV, and the intercept
%     angle is less than or equal to a specified value. This limits the intercept
%     angle even when the UAV is within L2 of the path.
%     See L2PlusWP1.m for details
%
%         INPUTS
%             wp0     Waypoint 0 position in North-East-Down meters
%             wp1     Waypoint 1 position in North-East-Down meters
%             Puav    Position of UAV in North-East-Down meters
%             Vxyz    Inertial velocity in North-East-Down meters
%
%         PARAMETERS
%             switchDistance distance from wp1 to switch to WP2
%             tanIntercept  tangent of intercept angle
%             MaxDwnPthStar L2 multiplier to determmine downpath aimpoint
%             Turn2Track    true to turn toward T1 instead of L2
%             InitialPoint  true if no line tracking at first--fly direct to some initial point
%             IPStar        L2 multiplier to determing distance of IP from first wp0
%             Tstar         was called L2Base, time constant of response
%             
%         OUTPUTS
%             L2Vec   L2 vector toward aim point
%             as_c    commanded lateral acceleration
%             transition A boolean of whether to transition or not to the next waypoint

    persistent IPActive;  %true if flying toward IP
    persistent IP; % location of initial point

    persistent direction; % Keep track of the direction for patrol mode
    if isempty(direction)
        direction = int8(1);
    end
    
    % Track the last acceleration command so we can filter it.
    persistent last_as_c;
    if isempty(last_as_c)
        last_as_c = single(NaN);
    end
    
    Pwp1 = single(zeros(3,1));
    Pe_y = single(0);
    Dist2wp1 = single(0);
    MinDownPath = single(0);
    Dist2WPSwitch = single(0);
    L2DownPath = single(0);
    L2ToT = single(zeros(3,1));
    L2Vec = single(zeros(3,1));
    IP1 = single([0; 0;-999]); %signal for no IP
    as_c = single(0);
    transition = false;
    
    Pne = [Puav(1); Puav(2); 0]; %horizontal position
    Vne = [Vxyz(1); Vxyz(2); 0]; % horizontal velocity
    Groundspeed = norm(Vne);
    L2 = single(TStar*Groundspeed);
    
    % If neither waypoint is valid then don't do anything
    if ~wp0_found || ~wp1_found
        return;
    % Otherwise if the first two waypoints are next to each other (as is
    % common if the origin is the first waypoint and the boat latches that
    % as its start value) then transition to the next waypoint.
    elseif norm(wp1 - wp0) < switchDistance
        transition = true;
        
        % Also reset the acceleration command filter. This is necessary as
        % wp transitions may result in large swings. 
        last_as_c = single(NaN);
        return;
    end
    
    % Calculate N1 (right-hand orthogonal to T1) 
    % and T1 (unit vector pointing from wp0 to wp1)
    T1 = wp1 - wp0;
    T1 = T1/norm(T1);
    N1 = [-T1(2); T1(1); 0];
    
%     initialize the initial point
    if (isempty(IPActive))
        if (InitialPoint)
%             IP is set relative to the first "from" waypoint
            IPActive = -1;
            IP = [wp0(1); wp0(2); 0] - L2*IPStar*T1;
            
            if (norm(IP-Pne) < .001)
                IPActive = 0;
                IP = single([0; 0; -999]);
            end
        else
            IPActive = 0;
            IP = single([0; 0;-999]); %signal for no IP
        end
    end
    IP1 = IP;
    
    
    if (IPActive)
%         no line tracking, direct to IP
        L2Vec = L2*(IP - Pne)/norm(IP - Pne);
%         check to see if at the IP to terminate this mode
        if norm(IP - Pne) < .1*L2
            IPActive = 0;
        end
    else
         if (Pne(1) < 2)
             IP1 = IP1;
         end
%         IP not active, track WP lines
        Pwp1 = Pne - [wp1(1); wp1(2); 0]; % position of UAV relative to wp1
        Pe_y = single(Pwp1'*N1); % cross track error
        Dist2wp1 = -single(Pwp1'*T1); % distance to wp1

%         minimum down path distance for Aim Point intersection on T
%         is determined by the intercept angle but limited 
%         in case of very distant intecepts to MaxDwnPthStar*L2
        MinDownPath = single ( min( abs(Pe_y)/tanIntercept, MaxDwnPthStar*L2)); 
        Dist2WPSwitch = Dist2wp1 - switchDistance;
        if ( abs(Pe_y) > L2 )
    %             Make sure aimpoint is no closer to waypoint than calculated switch point.
            L2DownPath = MinDownPath;
        else
    %             within L2 of T and Dist2WPSwitch >= 0, but limit angle of L2 wrt T
            L2DownPath = (max(MinDownPath, (sqrt( L2^2 - Pe_y^2 ))));
        end
        
        if ( Dist2WPSwitch < 0 )
            transition = true;
        end
        
         % vector from Pwp1 to aim point on T1
         L2ToT = single(( Dist2wp1 - L2DownPath )*(-T1) - Pwp1);
         if (norm(L2ToT) < .001)
             L2Vec = L2*T1;
         else
            L2Vec = single(L2*( L2ToT/norm(L2ToT) )); % limit size to L2
         end
    %         L2Vec = L2ToT;
%         dummy statements
    end
    Zprod = single(Vxyz(1)*L2Vec(2) - Vxyz(2)*L2Vec(1)); %Z component of cross product
    
    % Now if the groundspeed of the vessel is zero, we make sure we don't
    % get a division-by-zero error and instead handle it gracefully.
    if Groundspeed > 0
        sinEta = single(Zprod/(Groundspeed*L2));
        as_c = single(2*Groundspeed^2/(L2)*sinEta);
    else
        sinEta = single(0.0);
        as_c = single(0.0);
    end

%         now override bank angle if heading in the wrong direction
    if ( Turn2Track && Dist2WPSwitch > 0 && ~IPActive ) 
%             turn to track not L2, gives min displacement from track
        if ( T1'*Vxyz < 0 )
            if ( Pe_y > 0 )
                as_c = single(99);
            else
                as_c = single(-99);
            end
        end
     else
%           turn toward L2, give min displacement toward wp0
        if ( L2Vec'*Vxyz < 0 )
            if ( sinEta < 0 )
                as_c = single(-99);
            else
                as_c = single(99);
            end
        end
    end
    
    % Now add a jump-filter on the commanded acceleration. We use a large
    % enough value here such that the acceleration cannot switch signs, but
    % will still work in low-speed situations.
    % Note: The following works with the initial value of NaN, how
    % convenient!
    if abs(as_c - last_as_c) > single(99)
        as_c = last_as_c;
    else
        last_as_c = as_c;
    end
end
